simulink model "engduino_drivers"  (R2014b)
settings: Solver=ode45  StartTime=0.0  StopTime=10.0  RelTol=1e-3
settings Model: Creator=Cosmin  LastModifiedBy=Cosmin
settings RTWCC: CustomSource=src/Engduino.h src/engduino_wrappers.cpp

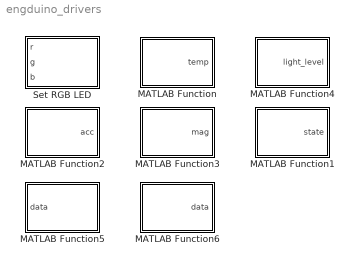
== system engduino_drivers ==
  MATLAB Function : MATLAB Function  LoadFcn=|  TreatAsAtomicUnit=on  mask(Thermistor){}
      | set_param(gcs, 'CustomSource', strjoin(unique([strsplit(get_param(gcs, 'CustomSource')) ...
      |  'src/engduino_wrappers.cpp' 'src/Engduino.h'])));
      mask help: Outputs the temperature in milli degrees celsius.
  MATLAB Function1 : MATLAB Function  LoadFcn=|  TreatAsAtomicUnit=on  mask(Button){}
      | set_param(gcs, 'CustomSource', strjoin(unique([strsplit(get_param(gcs, 'CustomSource')) ...
      |  'src/engduino_wrappers.cpp' 'src/Engduino.h'])));
      mask help: Outputs 1 if the button is pressed, 0 otherwise.
  MATLAB Function2 : MATLAB Function  LoadFcn=|  TreatAsAtomicUnit=on  mask(Accelerometer
Accelerometer){}
      | set_param(gcs, 'CustomSource', strjoin(unique([strsplit(get_param(gcs, 'CustomSource')) ...
      |  'src/engduino_wrappers.cpp' 'src/Engduino.h'])));
      mask help: Outputs a three components of the acceleration filed as a [x y z] vector.
  MATLAB Function3 : MATLAB Function  LoadFcn=|  TreatAsAtomicUnit=on  mask(Magnetometer){}
      | set_param(gcs, 'CustomSource', strjoin(unique([strsplit(get_param(gcs, 'CustomSource')) ...
      |  'src/engduino_wrappers.cpp' 'src/Engduino.h'])));
      mask help: Outputs a three components of the magnetic filed as a [x y z] vector.
  MATLAB Function4 : MATLAB Function  LoadFcn=|  TreatAsAtomicUnit=on  mask(Photodiode){}
      | set_param(gcs, 'CustomSource', strjoin(unique([strsplit(get_param(gcs, 'CustomSource')) ...
      |  'src/engduino_wrappers.cpp' 'src/Engduino.h'])));
      mask help: Outputs the light level as a uint16, in the range 0-1023.
  MATLAB Function5 : MATLAB Function  LoadFcn=|  TreatAsAtomicUnit=on  mask(IR Send){}
      | set_param(gcs, 'CustomSource', strjoin(unique([strsplit(get_param(gcs, 'CustomSource')) ...
      |  'src/engduino_wrappers.cpp' 'src/Engduino.h'])));
      mask help: Sends one byte at a time using the infrared transmitter.
  MATLAB Function6 : MATLAB Function  LoadFcn=|  TreatAsAtomicUnit=on  mask(IR Receive){}
      | set_param(gcs, 'CustomSource', strjoin(unique([strsplit(get_param(gcs, 'CustomSource')) ...
      |  'src/engduino_wrappers.cpp' 'src/Engduino.h'])));
      mask help: Receives one byte at a time using the infrared transmitter.
  Set RGB LED : MATLAB Function  LoadFcn=|  TreatAsAtomicUnit=on  mask(RGB LED){led_index=0}
      | set_param(gcs, 'CustomSource', strjoin(unique([strsplit(get_param(gcs, 'CustomSource')) ...
      |  'src/engduino_wrappers.cpp' 'src/Engduino.h'])));
      mask prompts: led_index "LED index"
      mask help:
      | Control the Red, Green and Blue color values of the LED specified by the LED index parameter.
      | Both the LED index and the three color values are of type uint8 and must be in the range 0-15.
      settings: AttributesFormatString=LED %<led_index>

== matlab function engduino_drivers/MATLAB Function1 ==
  data: state output
function state = button()

state = 0;

if strcmp(coder.target, 'rtw')
    state = coder.ceval('button_wrapper');
end

== matlab function engduino_drivers/MATLAB Function ==
  data: temp output
function temp = thermistor()

temp = 0.0;

if strcmp(coder.target, 'rtw')
    temp = coder.ceval('thermistor_wrapper');
end

== matlab function engduino_drivers/Set RGB LED ==
  data: led_index parameter uint8 [0..15]; r input uint8 [0..15]; g input uint8 [0..15]; b input uint8 [0..15]
function rgb_led(led_index, r, g, b)

if strcmp(coder.target, 'rtw')
    coder.ceval('rgb_leds_wrapper', led_index, r, g, b);
end

== matlab function engduino_drivers/MATLAB Function2 ==
  data: acc output size=[1, 3]
function acc = accelerometer()

acc = [0.0 0.0 0.0];

if strcmp(coder.target, 'rtw')
    coder.ceval('accelerometer_wrapper', coder.ref(acc));
end

== matlab function engduino_drivers/MATLAB Function3 ==
  data: mag output size=[1, 3]
function mag = magnetometer()

mag = [0.0 0.0 0.0];

if strcmp(coder.target, 'rtw')
    coder.ceval('magnetometer_wrapper', coder.ref(mag));
end

== matlab function engduino_drivers/MATLAB Function4 ==
  data: light_level output
function light_level = photodiode()

light_level = 0.0;

if strcmp(coder.target, 'rtw')
    light_level = coder.ceval('photodiode_wrapper');
end

== matlab function engduino_drivers/MATLAB Function5 ==
  data: data input uint8
function ir_send(data)

if strcmp(coder.target, 'rtw')
    coder.ceval('ir_send_wrapper', data);
end

== matlab function engduino_drivers/MATLAB Function6 ==
  data: data output uint8
function data = ir_receive()

data = uint8(0);

if strcmp(coder.target, 'rtw')
    data = coder.ceval('ir_receive_wrapper');
end
